simulink model "Torque_on_hardware"  (R2023b)
settings: Solver=FixedStepAuto  StartTime=0.0  StopTime=30  RelTol=1e-3  EnableMultiTasking=on
values from neighbouring files (symbols this model uses):
  alpha = exp(-Tfs/Ts)    [torque.m]
  k = kt    (= 1.45433391507)    [torque.m]
  Ts = 0.005    [torque.m]
libraries: mbedblockslib x4, cstblocks x2, eeStairGenerator x1
settings Model: ExtModeTrigDuration=10  Creator=giova  LastModifiedBy=david
settings OptimizationCC: EnhancedBackFolding=on  PassReuseOutputArgsAs=Individual arguments  ZeroExternalMemoryAtStartup=off  ZeroInternalMemoryAtStartup=off  MaxStackSize=64  OptimizeBlockOrder=speed  DifferentSizesBufferReuse=on  OptimizationCustomize=off  EfficientTunableParamExpr=on
settings DebuggingCC: ParameterTunabilityLossMsg=error
settings HardwareCC: ProdBitPerPointer=32  ProdBitPerSizeT=32  ProdBitPerPtrDiffT=32  ProdLargestAtomicInteger=Long  ProdLargestAtomicFloat=Double  ProdWordSize=32  ProdLongLongMode=on  ProdHWDeviceType=ARM Compatible->ARM Cortex
settings SFSimCC: MATLABDynamicMemAlloc=off
settings RTWCC: Description=Embedded Coder  SystemTargetFile=ert.tlc  HardwareBoard=STM32 Nucleo F401RE  TemplateMakefile=ert_default_tmf  Toolchain=GNU Tools for ARM Embedded Processors
settings CodeAppCC: ForceParamTrailComments=on  IgnoreCustomStorageClasses=off  OperatorAnnotations=on  SimulinkDataObjDesc=on  SFDataObjDesc=on  InsertBlockDesc=on
settings ERTTargetCC: ExtModeTransport=3  ExtModeStaticAlloc=on  ExtModeStaticAllocSize=2000  ExtModeMexFile=ext_xcp  ExtModeIntrfLevel=Level2 - Open

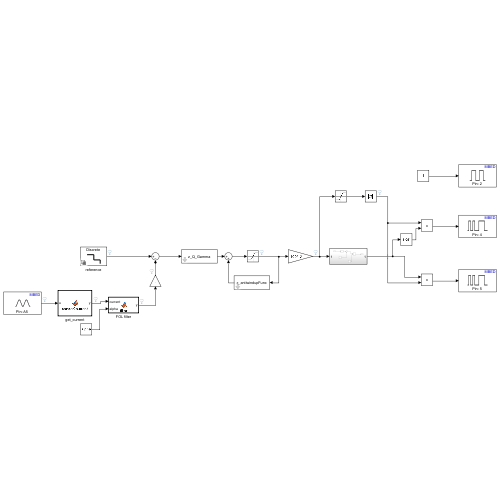
[thumbnail: Simulink's stored preview of the top-level diagram]
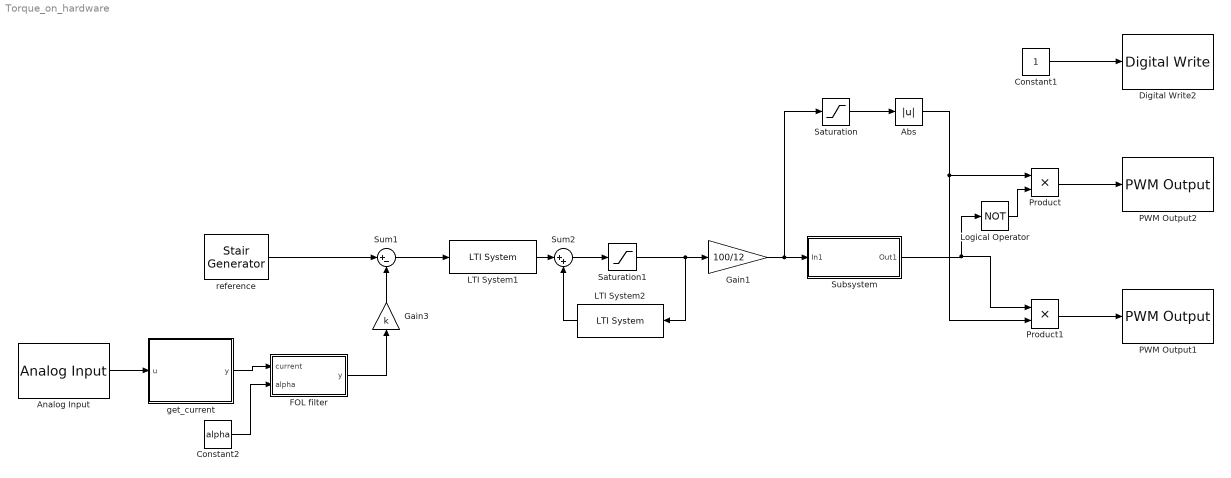
== system Torque_on_hardware ==
  Abs : Abs  SaturateOnIntegerOverflow=off
  Analog Input : mbedblockslib/Analog Input  Pin=A5  ReadResultsOnly=off  ConversionTriggerSource=Software  ExternalTriggerType=uint32( 0 )  OutputDataType=double  EnableConversionCompleteNotify=off  EnableOuputStatus=off  SampleTime=Ts
      settings: LibrarySourceBlock=stmnucleorootlib/Common/Analog Input
  Constant1 : Constant
  Constant2 : Constant  Value=alpha
  Digital Write2 : mbedblockslib/Digital Write  Pin=2  Direction=output
      settings: LibrarySourceBlock=stmnucleorootlib/Common/Digital Write
  FOL filter : MATLAB Function  TreatAsAtomicUnit=on
  Gain1 : Gain  Gain=100/12
  Gain3 : Gain  Gain=k
  LTI System1 : cstblocks/LTI System  sys=z_Q_Gamma  IC=[]  PadeOrder=0
  LTI System2 : cstblocks/LTI System  sys=z_antiwindupFunc  IC=[]  PadeOrder=0
  Logical Operator : Logic  Operator=NOT  AllPortsSameDT=off  OutDataTypeStr=boolean
  PWM Output1 : mbedblockslib/PWM Output  Pin=5  EnableInputFrequency=off  InitialFrequency=2000  InitialDutyCycle=50  NotificationType=None
      settings: LibrarySourceBlock=stmnucleorootlib/Common/PWM Output
  PWM Output2 : mbedblockslib/PWM Output  Pin=4  EnableInputFrequency=off  InitialFrequency=2000  InitialDutyCycle=50  NotificationType=None
      settings: LibrarySourceBlock=stmnucleorootlib/Common/PWM Output
  Product : Product
  Product1 : Product
  Saturation : Saturate  UpperLimit=100  LowerLimit=-100
  Saturation1 : Saturate  UpperLimit=12  LowerLimit=-12
  Subsystem : Subsystem
  Sum1 : Sum  Inputs=|+-
  Sum2 : Sum  Inputs=|++
  get_current : MATLAB Function  TreatAsAtomicUnit=on
  reference : eeStairGenerator/Stair Generator  LabelModeActiveChoice=Discrete  TimeInput=[0 11 21]  AmplitudeInput=[0.5 0.2 0]  SampleTime=Ts  RepeatPattern=off  OutDataTypeStr=double
      settings: LibrarySourceBlock=ee_sl_lib/General Control/Stair Generator
  wires:
  Sum1/1 -> LTI System1/1
  Gain3/1 -> Sum1/2
  Saturation/1 -> Abs/1
  Logical Operator/1 -> Product/2
  Constant1/1 -> Digital Write2/1
  Abs/1 -> Product1/2, Product/1
  Product1/1 -> PWM Output1/1
  Product/1 -> PWM Output2/1
  Gain1/1 -> Saturation/1, Subsystem/1(In1)
  Subsystem/1(Out1) -> Logical Operator/1, Product1/1
  FOL filter/1(y) -> Gain3/1
  Constant2/1 -> FOL filter/2(alpha)
  get_current/1(y) -> FOL filter/1(current)
  Analog Input/1 -> get_current/1(u)
  LTI System1/1 -> Sum2/1
  Sum2/1 -> Saturation1/1
  LTI System2/1 -> Sum2/2
  Saturation1/1 -> Gain1/1, LTI System2/1
  reference/1 -> Sum1/1

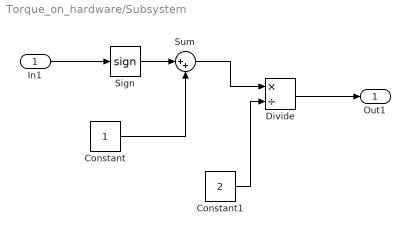
== system Torque_on_hardware/Subsystem ==
  In1 : Inport
  Constant : Constant
  Constant1 : Constant  Value=2
  Divide : Product  Inputs=*/
  Sign : Signum
  Sum : Sum  Inputs=|++
  Out1 : Outport
  wires:
  Constant/1 -> Sum/2
  In1/1 -> Sign/1
  Sign/1 -> Sum/1
  Sum/1 -> Divide/1
  Constant1/1 -> Divide/2
  Divide/1 -> Out1/1

== matlab function Torque_on_hardware/get_current ==
  data: u input; y output
function y  = sensor2current(u)
    v_input = u*3.3;
    current = (1/0.185)*(v_input-2.5530);
y = current

== matlab function Torque_on_hardware/FOL filter ==
  data: current input; y output; alpha input
function y = filter(current, alpha)
    persistent current_old current_filtered_old;

    if isempty(current_old)
        current_old = current;
        current_filtered_old = 0;
    else
        current_temp = current;
        current = alpha*current_filtered_old + (1 - alpha) *current_old;
        current_old = current_temp;
        current_filtered_old = current;
    end

y = current;
